simulink model "ERLE"  (R2013a)
settings: Solver=ode45  SolverMode=SingleTasking  StartTime=0.0  StopTime=10.0  RelTol=1e-3
values from neighbouring files (symbols this model uses):
  M = 0.95    [Variaveis.mat]
  T = 1    [Variaveis.mat]
settings Model: Creator=Afonso  LastModifiedBy=Élio
settings DataIOCC: SignalLoggingSaveFormat=ModelDataLogs
settings OptimizationCC: BlockReduction=off  BooleanDataType=off
settings DebuggingCC: SaveWithParameterizedLinksMsg=none  SignalResolutionControl=TryResolveAllWithWarning  SolverPrmCheckMsg=none  MultiTaskDSMMsg=warning  MultiTaskCondExecSysMsg=none  StrictBusMsg=None
settings HardwareCC: TargetUnknown=on
settings RTWCC: IncludeERTFirstTime=on

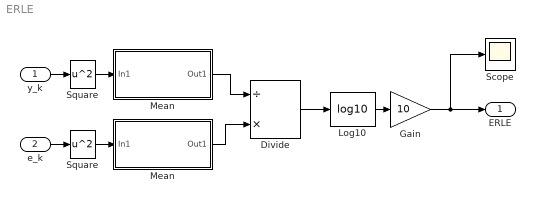
== system ERLE ==
  y_k : Inport
  e_k : Inport  Port=2
  Divide : Product  Inputs=/*
  Gain : Gain  Gain=10
  Log10 : Math  Operator=log10  SaturateOnIntegerOverflow=on
  Mean : Subsystem
  "Mean " : Subsystem
  Scope : Scope
  Square : Math  Operator=square  SaturateOnIntegerOverflow=on
  "Square " : Math  Operator=square  SaturateOnIntegerOverflow=on
  ERLE : Outport
  wires:
  e_k/1 -> "Square "/1
  y_k/1 -> Square/1
  "Square "/1 -> "Mean "/1(In1)
  "Mean "/1(Out1) -> Divide/2
  Log10/1 -> Gain/1
  Divide/1 -> Log10/1
  Gain/1 -> ERLE/1, Scope/1
  Mean/1(Out1) -> Divide/1
  Square/1 -> Mean/1(In1)

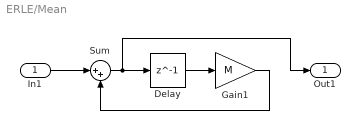
== system ERLE/Mean ==
  In1 : Inport
  Delay : Delay  DelayLength=1  SampleTime=T
  Gain1 : Gain  Gain=M
  Sum : Sum  Inputs=|++
  Out1 : Outport
  wires:
  Delay/1 -> Gain1/1
  Gain1/1 -> Sum/2
  In1/1 -> Sum/1
  Sum/1 -> Out1/1, Delay/1

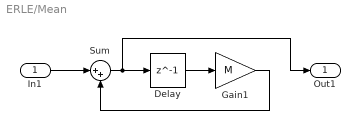
== system ERLE/Mean  ==
  In1 : Inport
  Delay : Delay  DelayLength=1  SampleTime=T
  Gain1 : Gain  Gain=M
  Sum : Sum  Inputs=|++
  Out1 : Outport
  wires:
  Delay/1 -> Gain1/1
  Gain1/1 -> Sum/2
  In1/1 -> Sum/1
  Sum/1 -> Out1/1, Delay/1
